simulink library "Pipe"  (Simulink 8.2)
settings: Solver=ode45  StartTime=0.0  StopTime=10.0  RelTol=1e-3
undefined symbols (not defined in the file): dia, height, nodes
libraries: carnot x1
settings Model: Creator=lena.frank  LastModifiedBy=drhf

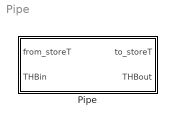
== system Pipe ==
  Pipe : Subsystem  mask(pipe connection to storage){h_in=0, h_out=1, nodes=nodes, hgt=height, dia=dia, dplin=0, dpqua=0}
      mask prompts: h_in "relative height of inlet"; h_out "relative height of outlet"; nodes "Number of nodes of storage (DO NOT CHANGE)"; hgt "Height vector (DO NOT CHANGE)"; dia "Diameter (DO NOT CHANGE)"; dplin "linear pressure drop"; dpqua "quadratic pressure drop"
      mask help:
      | The block transforms the incoming THV vector to a vector which the storage interprets as a flow into the storage fluid.
      | Give inlet- and outlet-height as a relative position from 0 (= bottom) to 1 (= top).
      mask init:
      | in = zeros(nodes,1);    % vector of length nodes
      | up = in;                % vector of length nodes
      | down = in;              % vector of length nodes
      | 
      | h_in = max(0,min(h_in,1));     % no nodes below 0
      | h_out = max(0,min(h_out,1));   % no nodes below 0
      | hgt = (h_out-h_in)*hgt;
      |  
      | inlet = max(ceil(h_in*nodes),1);    % inlet position
      | outlet = max(ceil(h_out*nodes),1);  % outlet position
      |  
      | in(inlet)=1;
      |  
      | idx_in_out = inlet:outlet;
      | if (inlet < outlet)         % if inlet below outlet
      |     up(inlet:outlet-1)=1;   % upwards
      | elseif (inlet > outlet)     % else if inlet above outlet
      |     down(outlet:inlet-1)=1; % downwards
      |     idx_in_out = outlet:inlet;
      | end
      mask Help: web(fullfile(path_carnot('help'),'StoragePorts_PipeConnections.html'),'-helpbrowser')
      mask Display: disp('Pipe')

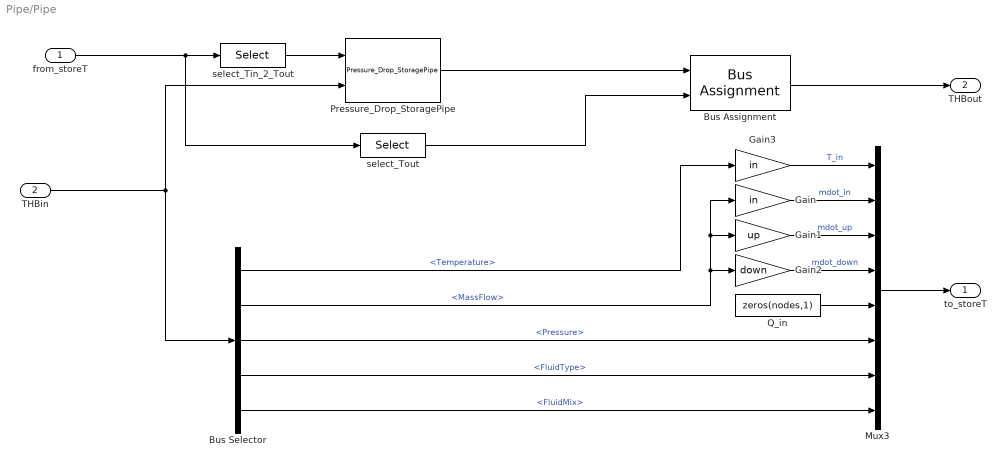
== system Pipe/Pipe ==
  from_storeT : Inport
  THBin : Inport  Port=2
  Bus Assignment : BusAssignment  AssignedSignals=Temperature
  Bus Selector : BusSelector  OutputSignals=Temperature,MassFlow,Pressure,FluidType,FluidMix
  Gain : Gain  Gain=in
  Gain1 : Gain  Gain=up
  Gain2 : Gain  Gain=down
  Gain3 : Gain  Gain=in
  Mux3 : Mux  Inputs=8
  Pressure_Drop_StoragePipe : carnot/Basic/Pressure_Drop/Pressure_Drop_StoragePipe  dia=dia  hgt=hgt
  Q_in : Constant  Value=zeros(nodes,1)
  select_Tin_2_Tout : Selector  InputPortWidth=nodes  IndexOptions=Index vector (dialog)  Indices=[idx_in_out]  OutputSizes=1
  select_Tout : Selector  InputPortWidth=nodes  IndexOptions=Index vector (dialog)  Indices=[outlet]  OutputSizes=1
  to_storeT : Outport
  THBout : Outport  Port=2
  wires:
  Pressure_Drop_StoragePipe/1 -> Bus Assignment/1
  from_storeT/1 -> select_Tout/1, select_Tin_2_Tout/1
  THBin/1 -> Pressure_Drop_StoragePipe/2, Bus Selector/1
  Bus Selector/4 -> Mux3/7  "<FluidType>"
  Bus Selector/3 -> Mux3/6  "<Pressure>"
  Bus Selector/2 -> Gain/1, Gain1/1, Gain2/1  "<MassFlow>"
  Bus Selector/1 -> Gain3/1  "<Temperature>"
  Gain/1 -> Mux3/2  "mdot_in"
  Gain1/1 -> Mux3/3  "mdot_up"
  Gain2/1 -> Mux3/4  "mdot_down"
  Mux3/1 -> to_storeT/1
  select_Tout/1 -> Bus Assignment/2
  Gain3/1 -> Mux3/1  "T_in"
  Q_in/1 -> Mux3/5
  Bus Assignment/1 -> THBout/1
  Bus Selector/5 -> Mux3/8  "<FluidMix>"
  select_Tin_2_Tout/1 -> Pressure_Drop_StoragePipe/1
